simulink model "mechanism"  (R2021a)
settings: Solver=VariableStepAuto  StartTime=0.0  StopTime=50  RelTol=1e-3
settings Model: Creator=hty  LastModifiedBy=hty

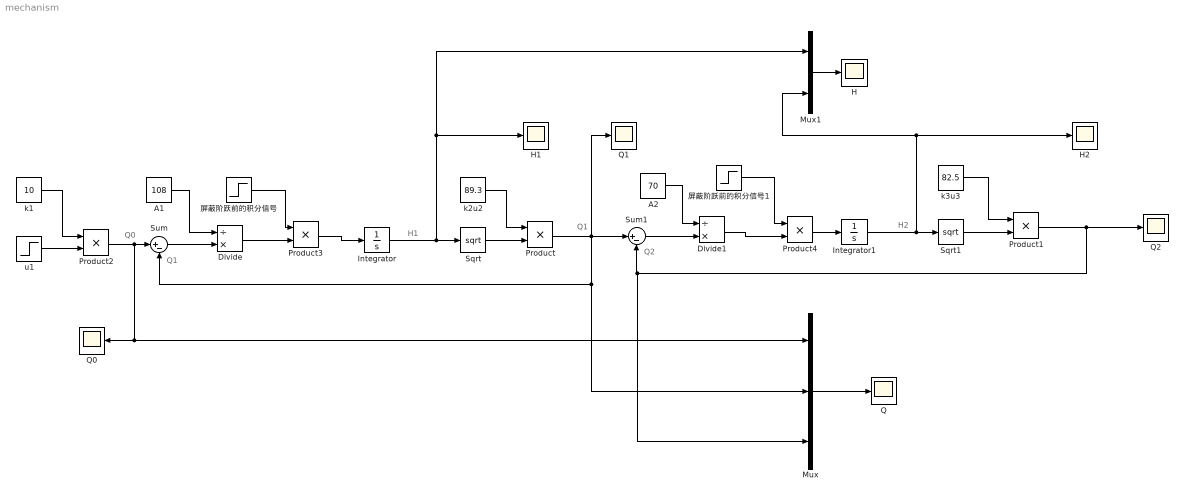
== system mechanism ==
  note: Q0
  note: H1
  note: Q1
  note: H2
  note: Q2
  note: Q1
  A1 : Constant  Value=108
  A2 : Constant  Value=70
  Divide : Product  Inputs=/*
  Divide1 : Product  Inputs=/*
  H : Scope
  H1 : Scope
  H2 : Scope
  Integrator : Integrator  InitialCondition=10
  Integrator1 : Integrator  InitialCondition=13
  Mux : Mux  Inputs=3
  Mux1 : Mux  Inputs=2
  Product{,1..4} (5 alike) : Product
  Q{,0..2} (4 alike) : Scope
  Sqrt : Sqrt  SaturateOnIntegerOverflow=on
  Sqrt1 : Sqrt  SaturateOnIntegerOverflow=on
  Sum : Sum  Inputs=|+-
  Sum1 : Sum  Inputs=|+-
  k1 : Constant  Value=10
  k2u2 : Constant  Value=89.3
  k3u3 : Constant  Value=82.5
  u1 : Step  Time=5  Before=28.2  After=28.2  SampleTime=0
  屏蔽阶跃前的积分信号 : Step  Time=5  SampleTime=0
  屏蔽阶跃前的积分信号1 : Step  Time=5  SampleTime=0
  wires:
  Sum/1 -> Divide/2
  A1/1 -> Divide/1
  Integrator/1 -> Mux1/1, H1/1, Sqrt/1
  Sqrt/1 -> Product/2
  k2u2/1 -> Product/1
  Product/1 -> Mux/2, Sum/2, Q1/1, Sum1/1
  Sum1/1 -> Divide1/2
  A2/1 -> Divide1/1
  Integrator1/1 -> Mux1/2, H2/1, Sqrt1/1
  Sqrt1/1 -> Product1/2
  k3u3/1 -> Product1/1
  Product1/1 -> Mux/3, Sum1/2, Q2/1
  u1/1 -> Product2/2
  k1/1 -> Product2/1
  Product2/1 -> Mux/1, Q0/1, Sum/1
  Divide/1 -> Product3/2
  Product3/1 -> Integrator/1
  屏蔽阶跃前的积分信号/1 -> Product3/1
  Product4/1 -> Integrator1/1
  Divide1/1 -> Product4/2
  屏蔽阶跃前的积分信号1/1 -> Product4/1
  Mux/1 -> Q/1
  Mux1/1 -> H/1
